simulink model "cstr5_sim_model"  (R2019b)
settings: Solver=VariableStepAuto  StartTime=0.0  StopTime=15  RelTol=1e-3
values from neighbouring files (symbols this model uses):
  sigma_v = [0; 0]    [cstr5_sim.m]    (also in cstr5_sim_EKF5.m = [20000; 0.2])
  sigma_w = (0.05 * x0).^2    [cstr5_sim_EKF5.m]
  Ts = diff(t_sim(1:2))    [cstr5_sim.m]    (also in cstr5_sim_EKF5.m; cstr5_sim_EKF7.m)
libraries: sharedTrackingLibrary x1
settings Model: Creator=billtubbs  LastModifiedBy=billtubbs

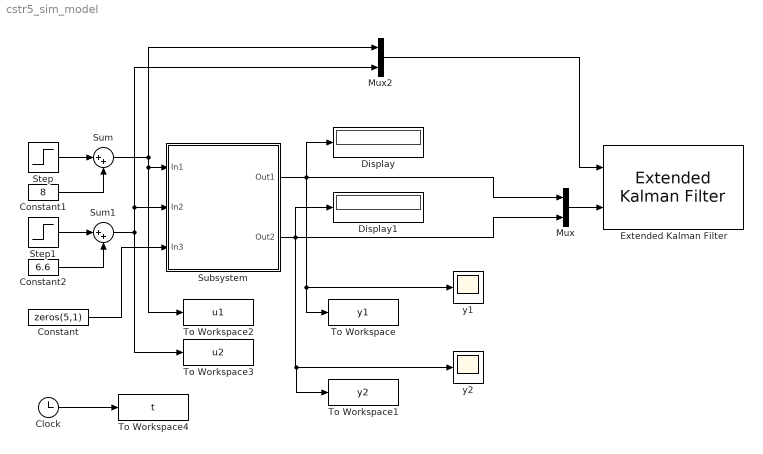
== system cstr5_sim_model ==
  Clock : Clock
  Constant : Constant  Value=zeros(5,1)  VectorParams1D=off
  Constant1 : Constant  Value=8
  Constant2 : Constant  Value=6.6
  Display : Display
  Display1 : Display
  Extended Kalman Filter : sharedTrackingLibrary/Extended Kalman Filter  StateTransitionFcn=cstr5_dynamics  HasStateTransitionJacobianFcn=off  StateTransitionJacobianFcn=cstr5_J  HasAdditiveProcessNoise=Additive  ProcessNoise=diag(sigma_w)  HasTimeVaryingProcessNoise=off  HasStateTransitionFcnExtraArgument=1  InitialState=InitialState  InitialStateCovariance=1  MeasurementFcn1=cstr5_measurements  HasMeasurementJacobianFcn1=off  MeasurementJacobianFcn1=cstr5_measJac  HasMeasurementEnablePort1=off  HasAdditiveMeasurementNoise1=Additive  MeasurementNoise1=diag(sigma_v)  HasTimeVaryingMeasurementNoise1=off  HasMeasurementFcnExtraArgument1=0  MeasurementFcn2=myMeasurementFcn  HasMeasurementJacobianFcn2=off  HasMeasurementEnablePort2=off  HasAdditiveMeasurementNoise2=Additive  MeasurementNoise2=1  HasTimeVaryingMeasurementNoise2=off  HasMeasurementFcnExtraArgument2=0  MeasurementFcn3=myMeasurementFcn  HasMeasurementJacobianFcn3=off  HasMeasurementEnablePort3=off  HasAdditiveMeasurementNoise3=Additive  MeasurementNoise3=1  HasTimeVaryingMeasurementNoise3=off  HasMeasurementFcnExtraArgument3=0  MeasurementFcn4=myMeasurementFcn  HasMeasurementJacobianFcn4=off  HasMeasurementEnablePort4=off  HasAdditiveMeasurementNoise4=Additive  MeasurementNoise4=1  HasTimeVaryingMeasurementNoise4=off  HasMeasurementFcnExtraArgument4=0  MeasurementFcn5=myMeasurementFcn  HasMeasurementJacobianFcn5=off  HasMeasurementEnablePort5=off  HasAdditiveMeasurementNoise5=Additive  MeasurementNoise5=1  HasTimeVaryingMeasurementNoise5=off  HasMeasurementFcnExtraArgument5=0  EnableMultirate=off  StateTransitionFcnSampleTime=1  MeasurementFcn1SampleTime=1  MeasurementFcn2SampleTime=1  MeasurementFcn3SampleTime=1  MeasurementFcn4SampleTime=1  MeasurementFcn5SampleTime=1  UseCurrentEstimator=on  OutputStateCovariance=off  DataType=double  SampleTime=Ts  NumberOfMeasurements=1
      settings: SourceProductName=Automated Driving Toolbox  SourceProductBaseCode=DR
  Mux : Mux  Inputs=2
  Mux2 : Mux  Inputs=2
  Step : Step  SampleTime=0
  Step1 : Step  Time=5  After=-1  SampleTime=0
  Subsystem : Subsystem
      mask Display:
      | disp('CSTR');
      | port_label('input', 1, 'Ci_in');
      | port_label('input', 2, 'Cm_in');
      | port_label('input', 3, 'w');
      | port_label('output', 1, 'D1/D0');
      | port_label('output', 2, 'T');
  Sum : Sum  Inputs=|++
  Sum1 : Sum  Inputs=|++
  To Workspace : ToWorkspace  VariableName=y1  SaveFormat=Timeseries  SampleTime=-1
  To Workspace1 : ToWorkspace  VariableName=y2  SaveFormat=Timeseries  SampleTime=-1
  To Workspace2 : ToWorkspace  VariableName=u1  SaveFormat=Timeseries  SampleTime=-1
  To Workspace3 : ToWorkspace  VariableName=u2  SaveFormat=Timeseries  SampleTime=-1
  To Workspace4 : ToWorkspace  VariableName=t  SaveFormat=Timeseries  SampleTime=-1
  y1 : Scope
  y2 : Scope
  wires:
  Constant1/1 -> Sum/2
  Step/1 -> Sum/1
  Step1/1 -> Sum1/1
  Constant2/1 -> Sum1/2
  Subsystem/2(Out2) -> Mux/2, To Workspace1/1, y2/1, Display1/1
  Subsystem/1(Out1) -> Mux/1, Display/1, To Workspace/1, y1/1
  Sum/1 -> To Workspace2/1, Subsystem/1(In1), Mux2/1
  Sum1/1 -> Mux2/2, Subsystem/2(In2), To Workspace3/1
  Constant/1 -> Subsystem/3(In3)
  Clock/1 -> To Workspace4/1
  Mux/1 -> Extended Kalman Filter/2
  Mux2/1 -> Extended Kalman Filter/1

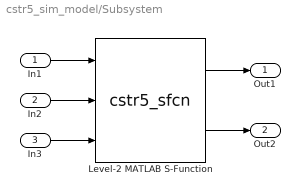
== system cstr5_sim_model/Subsystem ==
  In1 : Inport
  In2 : Inport  Port=2
  In3 : Inport  Port=3
  Level-2 MATLAB S-Function : M-S-Function  FunctionName=cstr5_sfcn
  Out1 : Outport
  Out2 : Outport  Port=2
  wires:
  In3/1 -> Level-2 MATLAB S-Function/3
  In2/1 -> Level-2 MATLAB S-Function/2
  Level-2 MATLAB S-Function/1 -> Out1/1
  Level-2 MATLAB S-Function/2 -> Out2/1
  In1/1 -> Level-2 MATLAB S-Function/1
